simulink library "rappid_564xl_ec_toolbox"  (R2016b)
(part 5 of 6)

      mask Help: web([rappid_block_help,filesep,'eTimer_preload.htm']);
      mask TypeOptions SubModule: 0 | 1 | 2
      mask TypeOptions Timerchan: 0 | 1 | 2 | 3 | 4 | 5
      mask Display:
      | disp(st);
      | port_label('input',1,'CNT');
      | port_label('input',2,'COMP1');
      | port_label('input',3,'COMP2')
